simulink model "Adaptive_Kalman_on_quad"  (R2015a)
settings: Solver=ode45  StartTime=0.0  StopTime=90  RelTol=1e-3
libraries: simulink x12, commnoisgen2 x7
settings Model: SimulationMode=accelerator  Creator=Oussama  LastModifiedBy=Oussama
settings OptimizationCC: EfficientMapNaN2IntZero=off
settings HardwareCC: TargetLongLongMode=on  TargetIntDivRoundTo=Zero  TargetEndianess=LittleEndian  TargetHWDeviceType=MATLAB Host  ProdEqTarget=off
settings CodeAppCC: MaxIdLength=128
settings GRTTargetCC: CombineOutputUpdateFcns=off  GRTInterface=on

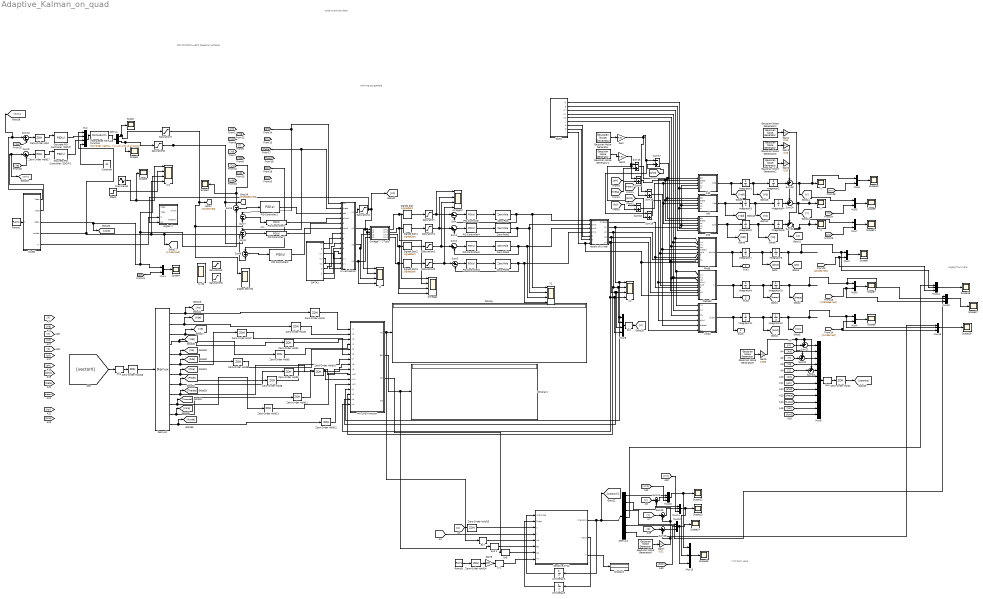
== system Adaptive_Kalman_on_quad ==
  note: angles from here
  note: XYZ from Here
  note: working acceptable
  note: used to extract data
  note: PID CONTROL+EKF based on Jacobian
  note: d25
  1x1 : Reshape  OutputDimensionality=Customize
  2x2 : Reshape  OutputDimensionality=Customize  OutputDimensions=[4,1]
  5x1 : Reshape  OutputDimensionality=Customize  OutputDimensions=[12,1]
  5x2 1 : Reshape  OutputDimensionality=Customize  OutputDimensions=[12,4]
  5x4 : Reshape  OutputDimensionality=Customize  OutputDimensions=[12,1]
  5x6 : Reshape  OutputDimensionality=Customize  OutputDimensions=[12,12]
  5x7 : Reshape  OutputDimensionality=Customize  OutputDimensions=[12,12]
  Constant : Constant  Value=10
  DATA : MATLAB Function  TreatAsAtomicUnit=on
  DATA1 : MATLAB Function  TreatAsAtomicUnit=on
  Demux : Demux  Outputs=2
  Demux1 : Demux  Outputs=12
  Demux2 : Demux  Outputs=12
  Discrete PID Controller (2DOF) : simulink/Continuous/PID Controller (2DOF)  Controller=PID  TimeDomain=Discrete-time  SampleTime=0.01  IntegratorMethod=Forward Euler  FilterMethod=Forward Euler  Form=Parallel  UseFilter=on  ControllerParametersSource=internal  P=0.4  I=0.3  D=3.2  N=100  b=1  c=1  InitialConditionSource=internal  InitialConditionForIntegrator=0  InitialConditionForFilter=0  ExternalReset=none  LimitOutput=off  UpperSaturationLimit=inf  LowerSaturationLimit=-inf  LinearizeAsGain=off  AntiWindupMode=none  Kb=1  TrackingMode=off  Kt=1  PParamMin=[]  PParamMax=[]  IParamMin=[]  IParamMax=[]  DParamMin=[]  DParamMax=[]  NParamMin=[]  NParamMax=[]  bParamMin=[]  bParamMax=[]  cParamMin=[]  cParamMax=[]  KbParamMin=[]  KbParamMax=[]  KtParamMin=[]  KtParamMax=[]  POutMin=[]  POutMax=[]  IOutMin=[]  IOutMax=[]  DOutMin=[]  DOutMax=[]  NOutMin=[]  NOutMax=[]  bOutMin=[]  bOutMax=[]  cOutMin=[]  cOutMax=[]  KbOutMin=[]  KbOutMax=[]  KtOutMin=[]  KtOutMax=[]  IntegratorOutMin=[]  IntegratorOutMax=[]  FilterOutMin=[]  FilterOutMax=[]  SumOutMin=[]  SumOutMax=[]  Sum1OutMin=[]  Sum1OutMax=[]  Sum2OutMin=[]  Sum2OutMax=[]  Sum3OutMin=[]  Sum3OutMax=[]  SumI1OutMin=[]  SumI1OutMax=[]  SumI2OutMin=[]  SumI2OutMax=[]  SumI3OutMin=[]  SumI3OutMax=[]  SumDOutMin=[]  SumDOutMax=[]  SaturationOutMin=[]  SaturationOutMax=[]  IntegratorContinuousStateAttributes=''  IntegratorStateMustResolveToSignalObject=off  IntegratorRTWStateStorageClass=Auto  FilterContinuousStateAttributes=''  FilterStateMustResolveToSignalObject=off  FilterRTWStateStorageClass=Auto  DifferentiatorICPrevScaledInput=0  DifferentiatorOutMin=[]  DifferentiatorOutMax=[]
  Discrete PID Controller (2DOF)1 : simulink/Continuous/PID Controller (2DOF)  Controller=PID  TimeDomain=Discrete-time  SampleTime=0.01  IntegratorMethod=Forward Euler  FilterMethod=Forward Euler  Form=Parallel  UseFilter=on  ControllerParametersSource=internal  P=0.7  I=0.5  D=1  N=100  b=1  c=1  InitialConditionSource=internal  InitialConditionForIntegrator=0  InitialConditionForFilter=0  ExternalReset=none  LimitOutput=off  UpperSaturationLimit=inf  LowerSaturationLimit=-inf  LinearizeAsGain=off  AntiWindupMode=none  Kb=1  TrackingMode=off  Kt=1  PParamMin=[]  PParamMax=[]  IParamMin=[]  IParamMax=[]  DParamMin=[]  DParamMax=[]  NParamMin=[]  NParamMax=[]  bParamMin=[]  bParamMax=[]  cParamMin=[]  cParamMax=[]  KbParamMin=[]  KbParamMax=[]  KtParamMin=[]  KtParamMax=[]  POutMin=[]  POutMax=[]  IOutMin=[]  IOutMax=[]  DOutMin=[]  DOutMax=[]  NOutMin=[]  NOutMax=[]  bOutMin=[]  bOutMax=[]  cOutMin=[]  cOutMax=[]  KbOutMin=[]  KbOutMax=[]  KtOutMin=[]  KtOutMax=[]  IntegratorOutMin=[]  IntegratorOutMax=[]  FilterOutMin=[]  FilterOutMax=[]  SumOutMin=[]  SumOutMax=[]  Sum1OutMin=[]  Sum1OutMax=[]  Sum2OutMin=[]  Sum2OutMax=[]  Sum3OutMin=[]  Sum3OutMax=[]  SumI1OutMin=[]  SumI1OutMax=[]  SumI2OutMin=[]  SumI2OutMax=[]  SumI3OutMin=[]  SumI3OutMax=[]  SumDOutMin=[]  SumDOutMax=[]  SaturationOutMin=[]  SaturationOutMax=[]  IntegratorContinuousStateAttributes=''  IntegratorStateMustResolveToSignalObject=off  IntegratorRTWStateStorageClass=Auto  FilterContinuousStateAttributes=''  FilterStateMustResolveToSignalObject=off  FilterRTWStateStorageClass=Auto  DifferentiatorICPrevScaledInput=0  DifferentiatorOutMin=[]  DifferentiatorOutMax=[]
  Display : Display
  Display1 : Display
  Display2 : Display
  Gain : Gain  Gain=0.01
  Gain1 : Gain  Gain=0.01
  Gain2 : Gain  Gain=0.03
  Gain3 : Gain  Gain=0.03
  Gain4 : Gain  Gain=0.03
  Gain5 : Gain  Gain=0.005
  Gain6 : Gain  Gain=100
  Gain7 : Gain  Gain=0.01
  Gaussian Noise Generator : commnoisgen2/Gaussian Noise Generator  m=0  d=1  s=41  Ts=0.02  frameBased=off  sampPerFrame=1  orient=off  outDataType=double
  Gaussian Noise Generator1 : commnoisgen2/Gaussian Noise Generator  m=0  d=1  s=41  Ts=0.02  frameBased=off  sampPerFrame=1  orient=off  outDataType=double
  Gaussian Noise Generator2 : commnoisgen2/Gaussian Noise Generator  m=0.3  d=1  s=41  Ts=5  frameBased=off  sampPerFrame=1  orient=off  outDataType=double
  Gaussian Noise Generator3 : commnoisgen2/Gaussian Noise Generator  m=0.3  d=1  s=41  Ts=2.5  frameBased=off  sampPerFrame=1  orient=off  outDataType=double
  Gaussian Noise Generator4 : commnoisgen2/Gaussian Noise Generator  m=0.3  d=1  s=41  Ts=3.5  frameBased=off  sampPerFrame=1  orient=off  outDataType=double
  Gaussian Noise Generator5 : commnoisgen2/Gaussian Noise Generator  m=0  d=0.02  s=41  Ts=0.005  frameBased=off  sampPerFrame=1  orient=off  outDataType=double
  Gaussian Noise Generator6 : commnoisgen2/Gaussian Noise Generator  m=0  d=0.02  s=41  Ts=0.005  frameBased=off  sampPerFrame=1  orient=off  outDataType=double
  Integrator{1..12} (12 alike) : Integrator
  Interpreted MATLAB Function : MATLABFcn  MATLABFcn=fsolve(@(x)attitudes3(x,u(1),u(2),u(3),u(4)),[0,0])  OutputDimensions=2
  Iterative KF12 : MATLAB Function  TreatAsAtomicUnit=on
  MATLAB Function : MATLAB Function  TreatAsAtomicUnit=on
  Mux : Mux
  Mux{1..7} (7 alike) : Mux  Inputs=2
  Mux{10..16} (7 alike) : Mux  Inputs=3
  Mux8 : Mux  Inputs=12
  Mux9 : Mux
  Omega i ^2  calc : MATLAB Function  TreatAsAtomicUnit=on
  Omegas : Scope  NumInputPorts=4
      settings: YMin=-5~-5~-5~-5  YMax=5~5~5~5  SaveName=ScopeData3
  PID Controller{,4..6} (4 alike) : simulink/Continuous/PID Controller  Controller=PID  TimeDomain=Continuous-time  SampleTime=-1  IntegratorMethod=Forward Euler  FilterMethod=Forward Euler  Form=Parallel  UseFilter=on  ControllerParametersSource=internal  P=0.696663945518539  I=69.3627675374527  D=0.000480635781112464  N=569.937710840054  InitialConditionSource=internal  InitialConditionForIntegrator=0  InitialConditionForFilter=0  ExternalReset=none  LimitOutput=off  UpperSaturationLimit=+12  LowerSaturationLimit=-12  LinearizeAsGain=on  AntiWindupMode=clamping  Kb=1  TrackingMode=off  Kt=1  PParamMin=[]  PParamMax=[]  IParamMin=[]  IParamMax=[]  DParamMin=[]  DParamMax=[]  NParamMin=[]  NParamMax=[]  KbParamMin=[]  KbParamMax=[]  KtParamMin=[]  KtParamMax=[]  POutMin=[]  POutMax=[]  IOutMin=[]  IOutMax=[]  DOutMin=[]  DOutMax=[]  NOutMin=[]  NOutMax=[]  KbOutMin=[]  KbOutMax=[]  KtOutMin=[]  KtOutMax=[]  IntegratorOutMin=[]  IntegratorOutMax=[]  FilterOutMin=[]  FilterOutMax=[]  SumOutMin=[]  SumOutMax=[]  SumI1OutMin=[]  SumI1OutMax=[]  SumI2OutMin=[]  SumI2OutMax=[]  SumI3OutMin=[]  SumI3OutMax=[]  SumDOutMin=[]  SumDOutMax=[]  SaturationOutMin=[]  SaturationOutMax=[]  IntegratorContinuousStateAttributes=''  IntegratorStateMustResolveToSignalObject=off  IntegratorRTWStateStorageClass=Auto  FilterContinuousStateAttributes=''  FilterStateMustResolveToSignalObject=off  FilterRTWStateStorageClass=Auto  DifferentiatorICPrevScaledInput=0  DifferentiatorOutMin=[]  DifferentiatorOutMax=[]
  PID Controller1 : simulink/Continuous/PID Controller  Controller=PID  TimeDomain=Continuous-time  SampleTime=-1  IntegratorMethod=Forward Euler  FilterMethod=Forward Euler  Form=Parallel  UseFilter=on  ControllerParametersSource=internal  P=4  I=2  D=5  N=476.409993785115  InitialConditionSource=internal  InitialConditionForIntegrator=0  InitialConditionForFilter=0  ExternalReset=none  LimitOutput=off  UpperSaturationLimit=inf  LowerSaturationLimit=-inf  LinearizeAsGain=on  AntiWindupMode=none  Kb=1  TrackingMode=off  Kt=1  PParamMin=[]  PParamMax=[]  IParamMin=[]  IParamMax=[]  DParamMin=[]  DParamMax=[]  NParamMin=[]  NParamMax=[]  KbParamMin=[]  KbParamMax=[]  KtParamMin=[]  KtParamMax=[]  POutMin=[]  POutMax=[]  IOutMin=[]  IOutMax=[]  DOutMin=[]  DOutMax=[]  NOutMin=[]  NOutMax=[]  KbOutMin=[]  KbOutMax=[]  KtOutMin=[]  KtOutMax=[]  IntegratorOutMin=[]  IntegratorOutMax=[]  FilterOutMin=[]  FilterOutMax=[]  SumOutMin=[]  SumOutMax=[]  SumI1OutMin=[]  SumI1OutMax=[]  SumI2OutMin=[]  SumI2OutMax=[]  SumI3OutMin=[]  SumI3OutMax=[]  SumDOutMin=[]  SumDOutMax=[]  SaturationOutMin=[]  SaturationOutMax=[]  IntegratorContinuousStateAttributes=''  IntegratorStateMustResolveToSignalObject=off  IntegratorRTWStateStorageClass=Auto  FilterContinuousStateAttributes=''  FilterStateMustResolveToSignalObject=off  FilterRTWStateStorageClass=Auto  DifferentiatorICPrevScaledInput=0  DifferentiatorOutMin=[]  DifferentiatorOutMax=[]
  PID Controller2 : simulink/Continuous/PID Controller  Controller=PID  TimeDomain=Continuous-time  SampleTime=-1  IntegratorMethod=Forward Euler  FilterMethod=Forward Euler  Form=Parallel  UseFilter=on  ControllerParametersSource=internal  P=4.05643234281984  I=0.70959032661118  D=4.0859309721323  N=476.409993785115  InitialConditionSource=internal  InitialConditionForIntegrator=0  InitialConditionForFilter=0  ExternalReset=none  LimitOutput=off  UpperSaturationLimit=inf  LowerSaturationLimit=-inf  LinearizeAsGain=on  AntiWindupMode=none  Kb=1  TrackingMode=off  Kt=1  PParamMin=[]  PParamMax=[]  IParamMin=[]  IParamMax=[]  DParamMin=[]  DParamMax=[]  NParamMin=[]  NParamMax=[]  KbParamMin=[]  KbParamMax=[]  KtParamMin=[]  KtParamMax=[]  POutMin=[]  POutMax=[]  IOutMin=[]  IOutMax=[]  DOutMin=[]  DOutMax=[]  NOutMin=[]  NOutMax=[]  KbOutMin=[]  KbOutMax=[]  KtOutMin=[]  KtOutMax=[]  IntegratorOutMin=[]  IntegratorOutMax=[]  FilterOutMin=[]  FilterOutMax=[]  SumOutMin=[]  SumOutMax=[]  SumI1OutMin=[]  SumI1OutMax=[]  SumI2OutMin=[]  SumI2OutMax=[]  SumI3OutMin=[]  SumI3OutMax=[]  SumDOutMin=[]  SumDOutMax=[]  SaturationOutMin=[]  SaturationOutMax=[]  IntegratorContinuousStateAttributes=''  IntegratorStateMustResolveToSignalObject=off  IntegratorRTWStateStorageClass=Auto  FilterContinuousStateAttributes=''  FilterStateMustResolveToSignalObject=off  FilterRTWStateStorageClass=Auto  DifferentiatorICPrevScaledInput=0  DifferentiatorOutMin=[]  DifferentiatorOutMax=[]
  PID Controller3 : simulink/Continuous/PID Controller  Controller=PID  TimeDomain=Continuous-time  SampleTime=-1  IntegratorMethod=Forward Euler  FilterMethod=Forward Euler  Form=Parallel  UseFilter=on  ControllerParametersSource=internal  P=11  I=0.2  D=22  N=100  InitialConditionSource=internal  InitialConditionForIntegrator=0  InitialConditionForFilter=0  ExternalReset=none  LimitOutput=off  UpperSaturationLimit=inf  LowerSaturationLimit=-inf  LinearizeAsGain=on  AntiWindupMode=none  Kb=1  TrackingMode=off  Kt=1  PParamMin=[]  PParamMax=[]  IParamMin=[]  IParamMax=[]  DParamMin=[]  DParamMax=[]  NParamMin=[]  NParamMax=[]  KbParamMin=[]  KbParamMax=[]  KtParamMin=[]  KtParamMax=[]  POutMin=[]  POutMax=[]  IOutMin=[]  IOutMax=[]  DOutMin=[]  DOutMax=[]  NOutMin=[]  NOutMax=[]  KbOutMin=[]  KbOutMax=[]  KtOutMin=[]  KtOutMax=[]  IntegratorOutMin=[]  IntegratorOutMax=[]  FilterOutMin=[]  FilterOutMax=[]  SumOutMin=[]  SumOutMax=[]  SumI1OutMin=[]  SumI1OutMax=[]  SumI2OutMin=[]  SumI2OutMax=[]  SumI3OutMin=[]  SumI3OutMax=[]  SumDOutMin=[]  SumDOutMax=[]  SaturationOutMin=[]  SaturationOutMax=[]  IntegratorContinuousStateAttributes=''  IntegratorStateMustResolveToSignalObject=off  IntegratorRTWStateStorageClass=Auto  FilterContinuousStateAttributes=''  FilterStateMustResolveToSignalObject=off  FilterRTWStateStorageClass=Auto  DifferentiatorICPrevScaledInput=0  DifferentiatorOutMin=[]  DifferentiatorOutMax=[]
  PID Controller7 : simulink/Continuous/PID Controller  Controller=PID  TimeDomain=Continuous-time  SampleTime=-1  IntegratorMethod=Forward Euler  FilterMethod=Forward Euler  Form=Parallel  UseFilter=on  ControllerParametersSource=internal  P=12  I=0.2  D=20  N=100  InitialConditionSource=internal  InitialConditionForIntegrator=0  InitialConditionForFilter=0  ExternalReset=none  LimitOutput=off  UpperSaturationLimit=inf  LowerSaturationLimit=-inf  LinearizeAsGain=on  AntiWindupMode=none  Kb=1  TrackingMode=off  Kt=1  PParamMin=[]  PParamMax=[]  IParamMin=[]  IParamMax=[]  DParamMin=[]  DParamMax=[]  NParamMin=[]  NParamMax=[]  KbParamMin=[]  KbParamMax=[]  KtParamMin=[]  KtParamMax=[]  POutMin=[]  POutMax=[]  IOutMin=[]  IOutMax=[]  DOutMin=[]  DOutMax=[]  NOutMin=[]  NOutMax=[]  KbOutMin=[]  KbOutMax=[]  KtOutMin=[]  KtOutMax=[]  IntegratorOutMin=[]  IntegratorOutMax=[]  FilterOutMin=[]  FilterOutMax=[]  SumOutMin=[]  SumOutMax=[]  SumI1OutMin=[]  SumI1OutMax=[]  SumI2OutMin=[]  SumI2OutMax=[]  SumI3OutMin=[]  SumI3OutMax=[]  SumDOutMin=[]  SumDOutMax=[]  SaturationOutMin=[]  SaturationOutMax=[]  IntegratorContinuousStateAttributes=''  IntegratorStateMustResolveToSignalObject=off  IntegratorRTWStateStorageClass=Auto  FilterContinuousStateAttributes=''  FilterStateMustResolveToSignalObject=off  FilterRTWStateStorageClass=Auto  DifferentiatorICPrevScaledInput=0  DifferentiatorOutMin=[]  DifferentiatorOutMax=[]
  Phidd : MATLAB Function  TreatAsAtomicUnit=on
  Ramp1 : simulink/Sources/Ramp  slope=1  start=0  X0=0
  Ramp3 : simulink/Sources/Ramp  slope=1  start=0  X0=0
  Saturation : Saturate  UpperLimit=3000  LowerLimit=0
  Saturation1 : Saturate  UpperLimit=3000  LowerLimit=0
  Saturation2 : Saturate  UpperLimit=800  LowerLimit=0
  Saturation3 : Saturate  UpperLimit=800  LowerLimit=0
  Saturation4 : Saturate  UpperLimit=50  LowerLimit=1
  Saturation5 : Saturate  UpperLimit=+0.3  LowerLimit=-0.3
  Saturation6 : Saturate  UpperLimit=+0.3  LowerLimit=-0.3
  Saturation7 : Saturate  UpperLimit=0.4  LowerLimit=-0.4
  Saturation8 : Saturate  UpperLimit=0.4  LowerLimit=-0.41
  Scope{,1..2,4..18} (18 alike) : Scope
      Scope settings: TimeRange=10  YMin=0.00025  YMax=0.00325
      Scope10 settings: SaveName=xdata
      Scope11 settings: TimeRange=10  YMin=7.74  YMax=7.94  SaveName=zdata
      Scope12 settings: YMin=7.775  YMax=8.075  SaveName=theta1
      Scope13 settings: YMin=6.9  YMax=7.14  SaveName=theta2
      Scope14 settings: YMin=7.451  YMax=7.47  SaveName=theta3
      Scope15 settings: YMin=-15  YMax=15  SaveName=X3Y3Z3
      Scope16 settings: YMin=-0.4  YMax=0.6  SaveName=phi3
      Scope17 settings: YMin=-0.4  YMax=0.6  SaveName=theta3
      Scope18 settings: YMin=0  YMax=0.00175  SaveName=psi3
      Scope2 settings: SaveName=ScopeData8
      Scope4 settings: SaveName=ScopeData10
      Scope5 settings: SaveName=ScopeData11
      Scope6 settings: YMin=-0.4  YMax=0.6  SaveName=phi
      Scope7 settings: YMin=-0.5  YMax=0.4  SaveName=theta
      Scope8 settings: YMin=-0.015  YMax=0.02  SaveName=psi
      Scope9 settings: YMin=-8  YMax=12  SaveName=ydata
  Signed Sqrt{,1..3} (4 alike) : Sqrt  Operator=signedSqrt  SaturateOnIntegerOverflow=on
  Sine Wave1 : Sin  Amplitude=20  Frequency=0.05  SampleTime=0
  Step2 : Step  Time=0  After=0  SampleTime=0
  Sum{,1..3,9..10} (6 alike) : Sum  Inputs=|+-
  Sum{13..14,20..23} (6 alike) : Sum  Inputs=++|
  Sum{4..8,15..19} (10 alike) : Sum  Inputs=-+
  Sum24 : Sum  Inputs=|++
  Sum25 : Sum  Inputs=|++
  Sum26 : Sum  Inputs=|++
  Ui : Scope  NumInputPorts=4
      settings: YMin=-5~-5~-5~-5  YMax=5~5~5~5  SaveName=ScopeData15
  Ui calculation : MATLAB Function  TreatAsAtomicUnit=on
  Ui1 : Scope  NumInputPorts=4
      settings: YMin=-5~-5~-5~-5  YMax=5~5~5~5  SaveName=traj
  Unit Delay3 : UnitDelay  SampleTime=-1
  Unit Delay5 : UnitDelay  SampleTime=-1
  X : Scope
      settings: YMin=3.81  YMax=3.95  SaveName=ScopeData6
  X1 : Scope  NumInputPorts=4
      settings: YMin=-5~-5~-5~-5  YMax=5~5~5~5  SaveName=ScopeData16
  X2 : Scope  NumInputPorts=4
      settings: YMin=-5~-5~-5~-5  YMax=5~5~5~5  SaveName=ScopeData7
  Xdd : MATLAB Function  TreatAsAtomicUnit=on
  Y : Scope
      settings: YMin=-0.01095  YMax=-0.0103  SaveName=ScopeData5
  Ydd : MATLAB Function  TreatAsAtomicUnit=on
  "Z " : Scope
      settings: YMin=7.615  YMax=7.6215  SaveName=ScopeData2
  Zdd : MATLAB Function  TreatAsAtomicUnit=on
  Zero-Order Hold{,1..17} (18 alike) : ZeroOrderHold  SampleTime=0.01
  Zero-Pole{,1..3} (4 alike) : ZeroPole  Zeros=[]  Poles=[-22.5]  Gain=[509]
  angles 1 : MATLAB Function  TreatAsAtomicUnit=on
  angles desired : Scope  NumInputPorts=2
      settings: YMin=-5~-5  YMax=5~5  SaveName=traj1
  "hjsdfd " : MATLAB Function  TreatAsAtomicUnit=on
  ksidd : MATLAB Function  TreatAsAtomicUnit=on
  omegas2 : Scope  NumInputPorts=4
      settings: YMin=-5~-5~-5~-5  YMax=5~5~5~5  SaveName=ScopeData4
  recalc of Ui real : MATLAB Function  TreatAsAtomicUnit=on
  thetadd : MATLAB Function  TreatAsAtomicUnit=on
  "xy dd " : Scope  NumInputPorts=2
      settings: YMin=-5~-5  YMax=5~5  SaveName=traj2
  Out2 : Outport
  Out3 : Outport  Port=2
  Out4 : Outport  Port=3
  wires:
  Mux/1 -> Interpreted MATLAB Function/1
  Demux/1 -> Saturation7/1, Scope/1
  Demux/2 -> Saturation8/1, Scope1/1
  Interpreted MATLAB Function/1 -> Demux/1
  Zero-Pole/1 -> Sum/2, X1/1, recalc of Ui real/1(om1)
  Sum/1 -> PID Controller/1
  Saturation/1 -> omegas2/1, Sum/1
  PID Controller/1 -> Zero-Pole/1
  Zero-Pole1/1 -> Sum1/2, X1/2, recalc of Ui real/2(om2)
  Sum1/1 -> PID Controller4/1
  Saturation1/1 -> omegas2/2, Sum1/1
  PID Controller4/1 -> Zero-Pole1/1
  Zero-Pole2/1 -> Sum2/2, X1/3, recalc of Ui real/3(om3)
  Sum2/1 -> PID Controller5/1
  Saturation2/1 -> omegas2/3, Sum2/1
  PID Controller5/1 -> Zero-Pole2/1
  Zero-Pole3/1 -> Sum3/2, X1/4, recalc of Ui real/4(om4)
  Sum3/1 -> PID Controller6/1
  Saturation3/1 -> omegas2/4, Sum3/1
  PID Controller6/1 -> Zero-Pole3/1
  Signed Sqrt/1 -> Saturation/1
  Signed Sqrt1/1 -> Saturation1/1
  Signed Sqrt2/1 -> Saturation2/1
  Signed Sqrt3/1 -> Saturation3/1
  Saturation4/1 -> angles 1/4(U1), Ui/1, Omega i ^2  calc/1(u1), [U1]
  Ui calculation/2(u2) -> Ui/2, Omega i ^2  calc/2(u2)
  Ui calculation/4(u4) -> Ui/4, Omega i ^2  calc/4(u4)
  Xdd/1(Xdd) -> [Xdd], Integrator1/1
  Ydd/1(Ydd) -> [Ydd], Integrator3/1
  Zdd/1(Zdd) -> [zdd], Integrator5/1
  Phidd/1(phidd) -> Out2/1, Integrator7/1
  Integrator7/1 -> [phid], Integrator8/1
  thetadd/1(thetadd) -> Out3/1, Integrator9/1
  Integrator9/1 -> [thetad], Integrator10/1
  ksidd/1(ksidd) -> Out4/1, Integrator11/1
  Integrator11/1 -> [ksid], Integrator12/1
  Integrator8/1 -> Mux14/2, Mux2/1, [phi]
  DATA/1(m) -> Zdd/5(m), Ydd/5(m), Xdd/5(m)
  DATA/2(g) -> Zdd/6(g)
  DATA/3(Ixx) -> ksidd/1(Ixx), thetadd/1(Ixx), Phidd/1(Ixx)
  DATA/4(Iyy) -> Phidd/2(Iyy), ksidd/2(Iyy), thetadd/2(Iyy)
  DATA/5(Izz) -> thetadd/3(Izz), ksidd/3(Izz), Phidd/3(Izz)
  DATA/6(J) -> thetadd/7(J), Phidd/7(J)
  Sum15/1 -> Zdd/1(phi), Ydd/1(phi), Xdd/1(phi)
  Sum4/1 -> Zdd/2(theta), Ydd/2(theta), Xdd/2(theta)
  Sum16/1 -> Ydd/3(ksi), Zdd/3(ksi), Xdd/3(ksi)
  Sum18/1 -> Phidd/4(thetad), ksidd/5(thetad)
  Sum19/1 -> Phidd/5(ksid), thetadd/5(ksid)
  Sum17/1 -> ksidd/4(phid), thetadd/4(phid)
  recalc of Ui real/1(omega) -> thetadd/6(omega), Phidd/6(omega)
  DATA/7(b) -> recalc of Ui real/5(b)
  DATA/8(d) -> recalc of Ui real/6(d)
  DATA1/1(m) -> Ui calculation/7(m)
  DATA1/2(g) -> Ui calculation/8(g)
  DATA1/6(b) -> Ui calculation/9(b)
  DATA1/7(d) -> Ui calculation/10(d)
  DATA1/8(l) -> Ui calculation/11(l)
  DATA1/3(Ixx) -> Ui calculation/12(Ixx)
  DATA1/4(Iyy) -> Ui calculation/13(Iyy)
  DATA1/5(Izz) -> Ui calculation/14(Izz)
  recalc of Ui real/5(u4) -> MATLAB Function/16(u4), Mux9/4, X2/4, ksidd/6(u4)
  recalc of Ui real/4(u3) -> MATLAB Function/15(u3), Mux9/3, X2/3, thetadd/8(u3)
  recalc of Ui real/3(u2) -> Mux9/2, X2/2, MATLAB Function/14(u2), Phidd/8(u2)
  Ui calculation/3(u3) -> Ui/3, Omega i ^2  calc/3(u3)
  Omega i ^2  calc/1(om1) -> Omegas/1, Signed Sqrt/1
  Omega i ^2  calc/2(om2) -> Omegas/2, Signed Sqrt1/1
  Omega i ^2  calc/3(om3) -> Omegas/3, Signed Sqrt2/1
  Omega i ^2  calc/4(om4) -> Omegas/4, Signed Sqrt3/1
  Gain1/1 -> Sum16/1, Sum4/1, Sum15/1
  [phi] -> Sum15/2
  [theta] -> Sum4/2
  [ksi] -> Sum16/2
  Gain/1 -> Sum19/1, Sum17/1, Sum18/1
  [phid] -> Sum17/2
  [thetad] -> Sum18/2
  [ksid] -> Sum19/2
  recalc of Ui real/2(u1) -> MATLAB Function/13(u1), Mux9/1, X2/1, Zdd/4(u1), Ydd/4(u1), Xdd/4(u1)
  Integrator5/1 -> [zd], Integrator6/1
  Integrator3/1 -> [Yd], Integrator4/1
  Integrator1/1 -> [Xd], Integrator2/1
  DATA/9(l) -> Phidd/9(l), thetadd/9(l), recalc of Ui real/7(l)
  Ramp1/1 -> "hjsdfd "/1(t)
  "hjsdfd "/3(Zdes) -> [ZZZ], Mux1/1, Ui1/3, Sum5/2
  [Ze] -> Scope2/1, Sum5/1
  Sum5/1 -> PID Controller1/1
  [phi] -> Ui calculation/1(phi), Sum7/1
  [theta] -> Ui calculation/2(theta), Sum8/1
  Sum6/1 -> PID Controller2/1
  [ksi] -> Sum6/1
  PID Controller2/1 -> Ui calculation/6(ksidd)
  Sum7/1 -> PID Controller3/1
  Sum8/1 -> PID Controller7/1
  PID Controller7/1 -> Ui calculation/5(thetadd)
  PID Controller3/1 -> Ui calculation/4(phidd)
  Saturation7/1 -> angles desired/1, Sum7/2, [phidesired]
  "hjsdfd "/5(m) -> angles 1/3(m)
  Sine Wave1/1 -> Scope5/1, Ui1/1
  PID Controller1/1 -> Ui calculation/3(zdd)
  Ui calculation/1(u1) -> Saturation4/1
  [Ze] -> Mux1/2
  Mux1/1 -> Scope4/1
  Step2/1 -> Ui1/2
  [phidesired] -> Mux14/3, Mux2/2
  Mux2/1 -> Scope6/1
  Integrator10/1 -> [theta], Mux15/2, Mux3/1
  [thetadesired] -> Mux15/3, Mux3/2
  Mux3/1 -> Scope7/1
  Integrator12/1 -> [ksi], Mux16/2, Mux4/1
  [Ksidesired] -> Mux16/3, Mux4/2
  Mux4/1 -> Scope8/1
  "hjsdfd "/4(ksides) -> [Ksidesired], Sum6/2, Ui1/4, Mux/1
  Sum10/1 -> Zero-Order Hold/1
  Sum9/1 -> Zero-Order Hold17/1
  ? -> angles desired/2
  "hjsdfd "/1(Xdes) -> [XXX], Sum10/1
  [Xe] -> Sum10/2
  "hjsdfd "/2(Ydes) -> Sum9/1, [YYY]
  [Ye] -> Sum9/2
  Sum14/1 -> [Y], Mux5/1, Y/1
  [YYY] -> Mux5/2
  Mux5/1 -> Scope9/1
  Sum13/1 -> [X], Mux6/1, X/1
  [XXX] -> Mux6/2
  Mux6/1 -> Scope10/1
  Sum20/1 -> Mux7/1, "Z "/1, [Z]
  [ZZZ] -> Mux7/2
  Mux7/1 -> Scope11/1
  Discrete PID Controller (2DOF)/1 -> Mux/2
  Discrete PID Controller (2DOF)1/1 -> Mux/3
  Saturation8/1 -> [thetadesired], Sum8/2
  Constant/1 -> Mux/4
  Integrator2/1 -> Sum13/2
  Gain2/1 -> Sum13/1
  Gain3/1 -> Sum14/1
  Integrator4/1 -> Sum14/2
  Integrator6/1 -> Sum20/2
  Gain4/1 -> Sum20/1
  Mux9/1 -> 2x2/1
  2x2/1 -> [U]
  5x4/1 -> Zero-Order Hold2/1
  Mux8/1 -> 5x4/1
  [X] -> Sum21/2
  [Y] -> Sum22/2
  [Yd] -> Mux8/4
  [Z] -> Sum23/2
  [zd] -> Mux8/6
  [phi] -> Mux8/7
  [phid] -> Mux8/8
  [theta] -> Mux8/9
  [thetad] -> Mux8/10
  [ksi] -> Mux8/11
  [ksid] -> Mux8/12
  Zero-Order Hold2/1 -> [sensors]
  Demux2/1 -> [Xe], Zero-Order Hold1/1
  Demux2/2 -> [Xde], Zero-Order Hold3/1
  Demux2/3 -> [Ye], Zero-Order Hold4/1
  Demux2/4 -> [Yde], Zero-Order Hold5/1
  Demux2/5 -> [Ze], Zero-Order Hold6/1
  Demux2/6 -> [Zde], Zero-Order Hold7/1
  Demux2/8 -> [Phide], Zero-Order Hold9/1
  Demux2/9 -> [Therae], Zero-Order Hold10/1
  Demux2/10 -> [Therade], Zero-Order Hold13/1
  Demux2/11 -> [Ksie], Zero-Order Hold11/1
  Demux2/12 -> [Kside], Zero-Order Hold12/1
  Zero-Order Hold1/1 -> MATLAB Function/1(x1)
  Zero-Order Hold3/1 -> MATLAB Function/2(x2)
  Zero-Order Hold4/1 -> MATLAB Function/3(x3)
  Zero-Order Hold5/1 -> MATLAB Function/4(x4)
  Zero-Order Hold6/1 -> MATLAB Function/5(x5)
  Zero-Order Hold7/1 -> MATLAB Function/6(x6)
  Zero-Order Hold8/1 -> MATLAB Function/7(x7)
  Zero-Order Hold9/1 -> MATLAB Function/8(x8)
  Zero-Order Hold10/1 -> MATLAB Function/9(x9)
  Zero-Order Hold11/1 -> MATLAB Function/11(x11)
  Zero-Order Hold12/1 -> MATLAB Function/12(x12)
  Zero-Order Hold13/1 -> MATLAB Function/10(x10)
  MATLAB Function/1(Ad) -> 5x7/1, Display/1
  MATLAB Function/2(Bd) -> 5x2 1/1, Display1/1
  MATLAB Function/3(Cd) -> 5x6/1
  5x7/1 -> Iterative KF12/5(Ad)
  5x2 1/1 -> Iterative KF12/6(Bd)
  5x6/1 -> Iterative KF12/7(Cd)
  Iterative KF12/1(Xnewpos) -> [vectorX], Demux1/1, Unit Delay3/1
  Unit Delay3/1 -> Iterative KF12/1(Xnewneg)
  Iterative KF12/2(Ppos) -> Unit Delay5/1
  Unit Delay5/1 -> Iterative KF12/2(Pneg)
  Ramp3/1 -> Zero-Order Hold14/1
  Zero-Order Hold14/1 -> Gain6/1
  1x1/1 -> Iterative KF12/8(TT)
  Gain6/1 -> 1x1/1
  Iterative KF12/3(T) -> Display2/1
  Zero-Order Hold15/1 -> Iterative KF12/3(U)
  [U] -> Zero-Order Hold15/1
  [sensors] -> Iterative KF12/4(Y)
  Demux1/1 -> Mux10/1
  [X] -> Sum24/1
  Mux10/1 -> Mux13/1, Scope12/1
  Demux1/3 -> Mux11/1
  Sum25/1 -> Mux11/2
  Mux11/1 -> Mux13/2, Scope13/1
  Demux1/5 -> Mux12/1
  Sum26/1 -> Mux12/2
  Mux12/1 -> Mux13/3, Scope14/1
  Zero-Order Hold16/1 -> Demux2/1
  5x1/1 -> Zero-Order Hold16/1
  [vectorX] -> 5x1/1
  Mux13/1 -> Scope15/1
  Gaussian Noise Generator2/1 -> Gain2/1
  Gaussian Noise Generator3/1 -> Gain3/1
  Gaussian Noise Generator4/1 -> Gain4/1
  Gaussian Noise Generator/1 -> Gain/1
  Gaussian Noise Generator1/1 -> Gain1/1
  Demux2/7 -> [Phie], Zero-Order Hold8/1
  Zero-Order Hold/1 -> Discrete PID Controller (2DOF)/1
  Zero-Order Hold17/1 -> Discrete PID Controller (2DOF)1/1
  Gaussian Noise Generator5/1 -> Gain5/1
  Sum21/1 -> Mux8/1
  Gain5/1 -> Sum22/1, Sum23/1, Sum21/1
  [Xd] -> Mux8/2
  Sum22/1 -> Mux8/3
  Sum23/1 -> Mux8/5
  Gaussian Noise Generator6/1 -> Gain7/1
  Sum24/1 -> Mux10/2
  Gain7/1 -> Sum26/2, Sum25/2, Sum24/2
  [Y] -> Sum25/1
  [Z] -> Sum26/1
  [XXX] -> Mux10/3
  [YYY] -> Mux11/3
  [ZZZ] -> Mux12/3
  Demux1/7 -> Mux14/1
  Demux1/9 -> Mux15/1
  Demux1/11 -> Mux16/1
  Mux14/1 -> Scope16/1
  Mux15/1 -> Scope17/1
  Mux16/1 -> Scope18/1

== matlab function Adaptive_Kalman_on_quad/Ydd ==
  data: phi input; Ydd output; theta input; ksi input; u1 input; m input
function Ydd = fcn(phi,theta, ksi,u1,m)
m=1;

Ydd=(-cos(ksi)*sin(phi)+sin(ksi)*sin(theta)*cos(phi))*u1/m;

== matlab function Adaptive_Kalman_on_quad/Zdd ==
  data: phi input; Zdd output; theta input; ksi input; u1 input; m input; g input
function Zdd = fcn(phi,theta, ksi,u1,m,g)
m=1;
g=9.81;

Zdd=-g+(cos(theta)*cos(phi))*u1/m;

== matlab function Adaptive_Kalman_on_quad/DATA ==
  data: m output; g output; Ixx output; Iyy output; Izz output; J output; b output; d output; l output
function [m,g,Ixx,Iyy,Izz,J,b,d,l] = fcn
m=1;
g=9.81;

Ixx=1*0.008;
Iyy=1*0.008;
Izz=1*0.015;
b=0.0001;
d=0.000001;
l=0.25;
J=0.0001;

== matlab function Adaptive_Kalman_on_quad/Phidd ==
  data: Ixx input; Iyy input; phidd output; Izz input; thetad input; ksid input; omega input; J input; u2 input; l input
function phidd = fcn(Ixx,Iyy,Izz,thetad, ksid,omega,J,u2,l)


phidd=1/Ixx*((Iyy-Izz)*thetad*ksid-J*thetad*omega+l*u2);

== matlab function Adaptive_Kalman_on_quad/thetadd ==
  data: Ixx input; Iyy input; thetadd output; Izz input; phid input; ksid input; omega input; J input; u3 input; l input
function thetadd = fcn(Ixx,Iyy,Izz,phid, ksid,omega,J,u3,l)


thetadd=1/Iyy*((Izz-Ixx)*phid*ksid+J*phid*omega+l*u3);

== matlab function Adaptive_Kalman_on_quad/ksidd ==
  data: Ixx input; Iyy input; ksidd output; Izz input; phid input; thetad input; u4 input
function ksidd = fcn(Ixx,Iyy,Izz,phid, thetad,u4)


ksidd=1/Izz*((Ixx-Iyy)*phid*thetad+u4);

== matlab function Adaptive_Kalman_on_quad/Omega i ^2  calc ==
  data: u1 input; om1 output; u2 input; u3 input; u4 input; om2 output; om3 output; om4 output
function [om1,om2,om3,om4] = fcn(u1,u2,u3,u4)
%#codegen
b=0.0001;
d=0.000001;
l=0.25;
A=[ 1/(4*b),0, -1/(2*b*l), -1/(4*d);1/(4*b), -1/(2*b*l),0,  1/(4*d); 1/(4*b),  0,  1/(2*b*l), -1/(4*d);1/(4*b),1/(2*b*l), 0,  1/(4*d)];
B=A*[u1;u2;u3;u4];
%[om1;om2;om3;om4]
om1= B(1);
om2=B(2);
om3=B(3);
om4=B(4);

== matlab function Adaptive_Kalman_on_quad/Ui calculation ==
  data: phi input; theta input; zdd input; u1 output; phidd input; thetadd input; ksidd input; u2 output; u3 output; u4 output; m input; g input; b input; d input; l input; Ixx input; Iyy input; Izz input
function [u1,u2,u3,u4] = fcn(phi, theta ,zdd, phidd, thetadd,ksidd,m,g,b,d,l,Ixx,Iyy,Izz )
%#codegen
u1=0;
u2=0;
u3=0;
u4=0;
u1= (zdd+g)*m/(cos(theta)*cos(phi));
u2= phidd*Ixx;
u3= thetadd*Iyy;
u4= ksidd*Izz;
b;
d;
l;
m;
g;

% if theta ==pi/2
%     u1=100;
% else 
%     if phi==pi/2
%         u1=100;
%     else
%             
% u1= (zdd+g)*m/(cos(theta)*cos(phi));
% u2= phidd*Ixx;
% u3= thetadd*Iyy;
% u4= ksidd*Izz;
% b;
% d;
% l;
% m;
% g;
% 
%     end
% end

== matlab function Adaptive_Kalman_on_quad/Xdd ==
  data: phi input; Xdd output; theta input; ksi input; u1 input; m input
function Xdd = fcn(phi,theta, ksi,u1,m)


Xdd=(sin(ksi)*sin(phi)+cos(ksi)*sin(theta)*cos(phi))*u1/m;

== matlab function Adaptive_Kalman_on_quad/recalc of Ui real ==
  data: om1 input; omega output; om2 input; om3 input; om4 input; b input; d input; l input; u1 output; u2 output; u3 output; u4 output
function [omega, u1,u2,u3,u4] = fcn(om1,om2,om3,om4,b,d,l)


omega=-om1+om2-om3+om4;
u1=b*(om1^2+om2^2+om3^2+om4^2);
u2=l*b*(om4^2-om2^2);
u3=l*b*(om3^2-om1^2);
u4=d*(om4^2+om2^2-om1^2-om3^2);

== matlab function Adaptive_Kalman_on_quad/DATA1 ==
  data: m output; g output; Ixx output; Iyy output; Izz output; b output; d output; l output
function [m,g,Ixx,Iyy,Izz,b,d,l] = fcn
m=1;
g=9.81;

Ixx=1*0.008;
Iyy=1*0.008;
Izz=1*0.015;
b=0.0001;
d=0.000001;
l=0.25;
%J=0.0001;

== matlab function Adaptive_Kalman_on_quad/Iterative KF12 ==
  data: Xnewneg input; Pneg input; U input; Y input; Ad input; Bd input; Cd input; Xnewpos output; Ppos output; T output; TT input
function [Xnewpos,Ppos,T]   = fcn(Xnewneg,Pneg,U,Y,Ad,Bd,Cd,TT)
%%%%%%%%%%%%%%%%%%%%%%%%%%%%%%%%%%%%%%%%%%%%%%%%%%%%
Q=0.01*eye(12);   % process noise covariance
R=0.05*eye(12);    % Measurement noise covariance
I=eye(12);
G=eye(12);
H=zeros(12,12);
Xnewneg=Xnewneg+[0,0,0,0,0,0,0,0,0,0,0,0]';
%%%%%%%%%%%%%%%%%%%%%%%%%%%%%%%%%%%%%%%%%%%%%%%%%%%%
Keneg=zeros(12,12);
Xnewpos=[0,0,0,0,0,0,0,0,0,0,0,0]';
Ppos=zeros(12,12);

Keneg=Pneg*Cd'/(Cd*Pneg*Cd'+R);
Xnewpos=Xnewneg+Keneg*(Y-Cd*Xnewneg);
Ppos=(I-Keneg*Cd)*Pneg*(I-Keneg*Cd)'+ Keneg*R*Keneg';

Xnewpos=Ad*Xnewpos+Bd*U;
Ppos=Ad*Ppos*Ad'+ G*Q*G';
T=TT+1;

== matlab function Adaptive_Kalman_on_quad/hjsdfd  ==
  data: t input; Xdes output; Ydes output; Zdes output; ksides output; m output
function [Xdes,Ydes,Zdes,ksides,m] = fcn(t)

A=5;a=5;
B=10;b=4;
C=8;c=5;
Xdes=A*cos(a*0.070*t);
Ydes=B*sin(b*0.07*t);
Zdes=C*(1-exp(-5*0.070*t));
%#codegen
m=1;
%ksides=0.2*cos(0.1*time)-0.32*sin(0.2*time);
ksides=0;
%plot3(Xdes,Ydes,Zdes,'*')
%hold on
%grid on

== matlab function Adaptive_Kalman_on_quad/angles 1 ==
  data: Xdes input; phitrk output; Ydes input; m input; U1 input; thetatrk output
function [phitrk,thetatrk]  = fcn(Xdes,Ydes, m,U1)
%#codegen
if U1<=5
    phitrk=0;
else
    if (abs(Ydes*m/U1) >= 0.3)
        phitrk= -sign(Ydes*m/U1)*pi/10;
    else
    phitrk=-asin(Ydes*m/U1);
    end
end
%%%%%%%%%%%%%%%%%%
if U1<=5
    thetatrk=0;
elseif (abs( Xdes*m/(U1*cos(phitrk)) ) >= 0.3 )
        thetatrk = sign( Xdes*m/(U1*cos(phitrk)) )*pi/10 ;
    else
    thetatrk=asin(Xdes*m/(U1*cos(phitrk)) );
end

    
%%%%%%%%%%%%
if phitrk > pi/3
    phitrk=pi/3;
end
if phitrk < -pi/3
    phitrk=-pi/3;
end
%%%%%%%%%%%%%%%
if thetatrk > pi/3
    thetatrk=pi/3;
end
if thetatrk < -pi/3
    thetatrk=-pi/3;
end

== matlab function Adaptive_Kalman_on_quad/MATLAB Function ==
  data: x1 input; Ad output; x2 input; x3 input; x4 input; x5 input; x6 input; x7 input; x8 input; x9 input; x10 input; x11 input; x12 input; u1 input; u2 input; u3 input; u4 input; Bd output; Cd output; Dd output
function [Ad,Bd,Cd,Dd] = fcn(x1,x2,x3,x4,x5,x6,x7,x8,x9,x10,x11,x12,u1,u2,u3,u4)
%#codegen

Ac = [0 1 0 0 0 0 0 0 0 0 0 0;
0 0 0 0 0 0 u1*(cos(x7)*sin(x11)-cos(x11)*sin(x7)*sin(x9)) 0 u1*cos(x7)*cos(x9)*cos(x11) 0 u1*(cos(x11)*sin(x7)-cos(x7)*sin(x9)*sin(x11)) 0;
0 0 0 1 0 0 0 0 0 0 0 0;
0 0 0 0 0 0 -u1*(cos(x7)*cos(x11)+sin(x7)*sin(x9)*sin(x11)) 0 u1*cos(x7)*cos(x9)*sin(x11) 0 u1*(sin(x7)*sin(x11)+cos(x7)*cos(x11)*sin(x9)) 0;
0 0 0 0 0 1 0 0 0 0 0 0;
0 0 0 0 0 0 -u1*cos(x9)*sin(x7) 0 -u1*cos(x7)*sin(x9) 0 0 0;
0 0 0 0 0 0 0 1 0 0 0 0;
0 0 0 0 0 0 0 0 0 5/4-(7*x12)/8 0 -(7*x10)/8;
0 0 0 0 0 0 0 0 0 1 0 0;
0 0 0 0 0 0 0 (7*x12)/8+5/4 0 0 0 (7*x8)/8;
0 0 0 0 0 0 0 0 0 0 0 1;
0 0 0 0 0 0 0 0 0 0 0 0];
 
Bc = [0 0 0 0;
sin(x7)*sin(x11)+cos(x7)*cos(x11)*sin(x9) 0  0 0;
0 0 0 0;
cos(x7)*sin(x9)*sin(x11)-cos(x11)*sin(x7) 0 0 0;
0 0 0 0;
cos(x7)*cos(x9) 0 0 0;
0 0 0 0;
0 125 0 0;
0 0 0 0;
0 0 125 0;
0 0 0 0;
0 0 0 200/3]

Cc=eye(12);
Cd=Cc;
Dc=zeros(12,4)
Dd=Dc;
kk=exp([Ac Bc; zeros(12,12) zeros(12,4)]*0.01)-ones(24,16)+eye(24,16);

Ad=kk(1:12,1:12);
Bd=kk(1:12,13:16);
